simulink model "siso_sys"  (R2015a)
settings: Solver=ode45  SolverMode=SingleTasking  StartTime=0.0  StopTime=10.0  RelTol=1e-3
values from neighbouring files (symbols this model uses):
  A = dsys.a    [master_disc_Hinf_feedback.m]
  Ts = 0.001    [master_disc_Hinf_feedback.m]
undefined symbols (not defined in the file or in its folder): Ac, Bc, Bu, Cc, Cy, Dc, Dyw
settings Model: Creator=enrico-giordano  LastModifiedBy=enrico-giordano
settings OptimizationCC: BlockReduction=off  BooleanDataType=off
settings DebuggingCC: SaveWithParameterizedLinksMsg=none  UnderspecifiedInitializationDetection=Classic  MergeDetectMultiDrivingBlocksExec=none  SignalResolutionControl=TryResolveAllWithWarning
settings HardwareCC: TargetUnknown=on

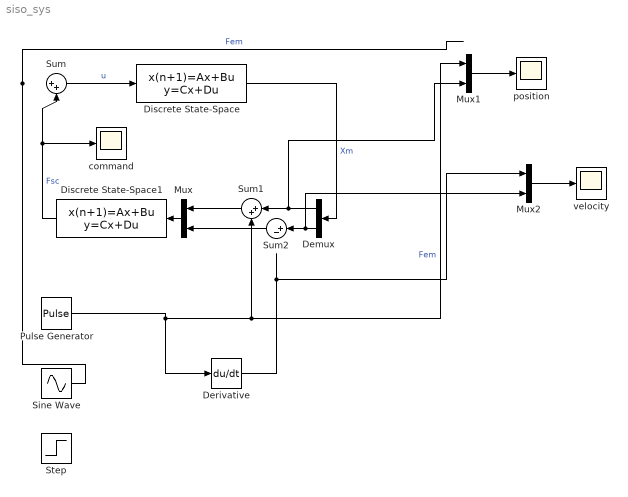
== system siso_sys ==
  Demux : Demux  Outputs=2
  Derivative : Derivative
  Discrete State-Space : DiscreteStateSpace  A=A  B=Bu  C=Cy  D=Dyw  SampleTime=Ts
  Discrete State-Space1 : DiscreteStateSpace  A=Ac  B=Bc  C=Cc  D=Dc  SampleTime=Ts
  Mux : Mux  Inputs=2
  Mux1 : Mux  Inputs=2
  Mux2 : Mux  Inputs=2
  Pulse Generator : DiscretePulseGenerator  PulseType=Time based  PulseWidth=50
  Sine Wave : Sin  Amplitude=10  SampleTime=0
  Step : Step  SampleTime=0
  Sum : Sum  Inputs=|++
  Sum1 : Sum  Inputs=|++
  Sum2 : Sum  Inputs=|+-
  command : Scope
      settings: TimeRange=10  YMin=-0.6000000000000001  YMax=0.2  SaveName=ScopeData2
  position : Scope
      settings: TimeRange=10  YMin=-0.6000000000000001  YMax=0.2
  velocity : Scope
      settings: TimeRange=10  YMin=-0.6000000000000001  YMax=0.2
  wires:
  Sum/1 -> Discrete State-Space/1  "u"
  Discrete State-Space/1 -> Demux/1  "Xm"
  Discrete State-Space1/1 -> Sum/2, command/1  "Fsc"
  Mux/1 -> Discrete State-Space1/1
  Demux/1 -> Mux1/2, Sum1/1
  Sum1/1 -> Mux/1
  Pulse Generator/1 -> Derivative/1, Mux1/1, Sum1/2  "Fem"
  Demux/2 -> Mux2/2, Sum2/1
  Mux1/1 -> position/1
  Sum2/1 -> Mux/2
  Derivative/1 -> Mux2/1
  Mux2/1 -> velocity/1
  Sine Wave/1 -> ?  "Fem"
